simulink library "cpcAux"  (R2016a)
settings: Solver=ode45  StartTime=0.0  StopTime=10.0  RelTol=1e-3
undefined symbols (not defined in the file): DiscIntNeverNeededParam, sMP
libraries: simulink x16, cpcAux x8
(part 1 of 2)
settings Model: Creator=lzaimog  LastModifiedBy=PLOCH37
settings DataIOCC: LimitDataPoints=on
settings DebuggingCC: AllowSymbolicDim=off

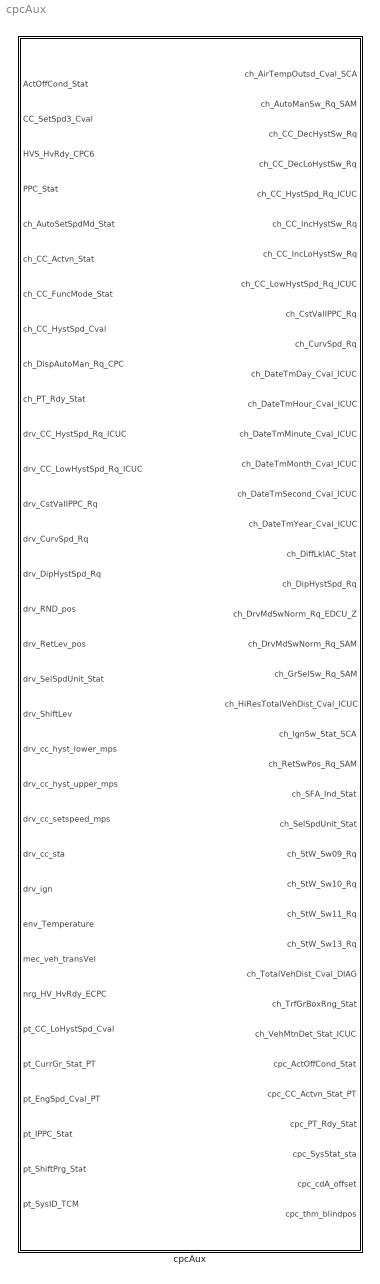
== system cpcAux ==
  cpcAux : Subsystem  TreatAsAtomicUnit=on  SystemSampleTime=0.1  mask{bShiftManual=sMP.ctrl.cpcAux.bShiftManual, s_shift_wait=sMP.ctrl.cpcAux.s_shift_wait, kmh_upshift=sMP.ctrl.cpcAux.kmh_upshift, kmh_downshift=sMP.ctrl.cpcAux.kmh_downshift, ShiftPrg=sMP.ctrl.cpcAux.ShiftPrg, CCFunc=sMP.ctrl.cpcAux.CCFunc, bCCbyPPC=sMP.ctrl.cpcAux.bCCbyPPC, x_id=sMP.ctrl.cpcAux.tfc_id, x_n=sMP.ctrl.cpcAux.tfc_gear, x_trqDistr=sMP.ctrl.cpcAux.tfc_trqDistribution, cdA_offset_sta=sMP.ctrl.cpcAux.cdA_offset_sta, cdA_offset_m2=sMP.ctrl.cpcAux.cdA_offset_m2, DateTmYear=sMP.ctrl.cpcAux.out.ch_DateTmYear_Cval_ICUC, DateTmMonth=sMP.ctrl.cpcAux.out.ch_DateTmMonth_Cval_ICUC, DateTmDay=sMP.ctrl.cpcAux.out.ch_DateTmDay_Cval_ICUC, DateTmHour=sMP.ctrl.cpcAux.out.ch_DateTmHour_Cval_ICUC, DateTmMinute=sMP.ctrl.cpcAux.out.ch_DateTmMinute_Cval_ICUC, DateTmSecond=sMP.ctrl.cpcAux.out.ch_DateTmSecond_Cval_ICUC}
      mask prompts: bShiftManual "Manual Shift [0,1]"; s_shift_wait "Wait Time between Shift [s]"; kmh_upshift "Upshift Speed [km/h]"; kmh_downshift "Downshift Speed [km/h]"; ShiftPrg "Drive program set by driver"; CCFunc "Function Mode [-]"; bCCbyPPC "CC controlled by IPPC [0,1]"; x_id "Type [-]"; x_n "Gear [-]"; x_trqDistr "Torque Distribution [%] (1x2)"; cdA_offset_sta "Blind position [-]"; cdA_offset_m2 "cd*A offset [m²]"; DateTmYear "Year"; DateTmMonth "Month"; DateTmDay "Day"; DateTmHour "Hour"; DateTmMinute "Minute"; DateTmSecond "Second"
      mask DialogControl DescTextVar Prompt: ICUC, SAM, ...

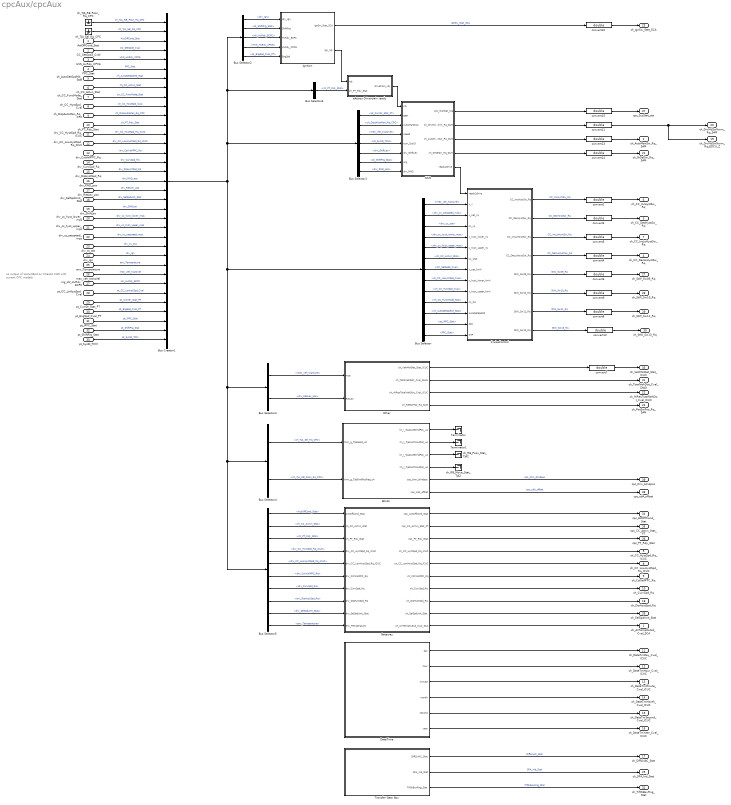
== system cpcAux/cpcAux ==
  note: no output of LoHystSpd on Chassis CAN
      | with current CPC models
  ActOffCond_Stat : Inport  OutDataTypeStr=double
  CC_SetSpd3_Cval : Inport  Port=2  OutDataTypeStr=double
  HVS_HvRdy_CPC6 : Inport  Port=3  OutDataTypeStr=double
  PPC_Stat : Inport  Port=4  OutDataTypeStr=double
  ch_AutoSetSpdMd_Stat : Inport  Port=5  OutDataTypeStr=double
  ch_CC_Actvn_Stat : Inport  Port=6  OutDataTypeStr=double
  ch_CC_FuncMode_Stat : Inport  Port=7  OutDataTypeStr=double
  ch_CC_HystSpd_Cval : Inport  Port=8  OutDataTypeStr=double
  ch_DispAutoMan_Rq_CPC : Inport  Port=9  OutDataTypeStr=double
  ch_PT_Rdy_Stat : Inport  Port=10  OutDataTypeStr=double
  drv_CC_HystSpd_Rq_ICUC : Inport  Port=11  OutDataTypeStr=double
  drv_CC_LowHystSpd_Rq_ICUC : Inport  Port=12  OutDataTypeStr=double
  drv_CstValIPPC_Rq : Inport  Port=13  OutDataTypeStr=double
  drv_CurvSpd_Rq : Inport  Port=14  OutDataTypeStr=double
  drv_DipHystSpd_Rq : Inport  Port=15  OutDataTypeStr=double
  drv_RND_pos : Inport  Port=16  OutDataTypeStr=double
  drv_RetLev_pos : Inport  Port=17  OutDataTypeStr=double
  drv_SelSpdUnit_Stat : Inport  Port=18  OutDataTypeStr=double
  drv_ShiftLev : Inport  Port=19  OutDataTypeStr=double
  drv_cc_hyst_lower_mps : Inport  Port=20  OutDataTypeStr=double
  drv_cc_hyst_upper_mps : Inport  Port=21  OutDataTypeStr=double
  drv_cc_setspeed_mps : Inport  Port=22  OutDataTypeStr=double
  drv_cc_sta : Inport  Port=23  OutDataTypeStr=double
  drv_ign : Inport  Port=24  OutDataTypeStr=double
  env_Temperature : Inport  Port=25  OutDataTypeStr=double
  mec_veh_transVel : Inport  Port=26  OutDataTypeStr=double
  nrg_HV_HvRdy_ECPC : Inport  Port=27  OutDataTypeStr=double
  pt_CC_LoHystSpd_Cval : Inport  Port=28  OutDataTypeStr=double
  pt_CurrGr_Stat_PT : Inport  Port=29  OutDataTypeStr=double
  pt_EngSpd_Cval_PT : Inport  Port=30  OutDataTypeStr=double
  pt_IPPC_Stat : Inport  Port=31  OutDataTypeStr=double
  pt_ShiftPrg_Stat : Inport  Port=32  OutDataTypeStr=double
  pt_SysID_TCM : Inport  Port=33  OutDataTypeStr=double
  Blinds : Subsystem  mask{cdA_offset_sta=cdA_offset_sta, cdA_offset_m2=cdA_offset_m2}
      mask prompts: cdA_offset_sta "Blind position [-]"; cdA_offset_m2 "cd*A offset [m²]"
      mask help:
      | Blind position [-]:
      | 0 - both open
      | 1 - bumper open, grill closed
      | 2 - bumper closed, grill open
      | 3 - both closed
  Bus Creator1 : BusCreator  Inputs=35
  Bus Selector : BusSelector  OutputSignals=mec_veh_transVel,drv_cc_setspeed_mps,drv_cc_sta,drv_cc_hyst_lower_mps,drv_cc_hyst_upper_mps,ch_CC_Actvn_Stat,CC_SetSpd3_Cval,pt_CC_LoHystSpd_Cval,ch_CC_HystSpd_Cval,ch_CC_FuncMode_Stat,ch_AutoSetSpdMd_Stat,pt_IPPC_Stat,PPC_Stat
  Bus Selector1 : BusSelector  OutputSignals=pt_CurrGr_Stat_PT,ch_DispAutoMan_Rq_CPC,mec_veh_transVel,pt_SysID_TCM,drv_ShiftLev,pt_ShiftPrg_Stat,drv_RND_pos
  Bus Selector2 : BusSelector  OutputSignals=drv_ign,pt_ShiftPrg_Stat,HV_HvRdy_ECPC,HVS_HvRdy_CPC6,pt_EngSpd_Cval_PT
  Bus Selector3 : BusSelector  OutputSignals=mec_veh_transVel,drv_RetLev_pos
  Bus Selector4 : BusSelector  OutputSignals=ch_TJA_Sel_Rq_CPC,ch_TJA_RB_Posn_Rq_CPC
  Bus Selector5 : BusSelector  OutputSignals=ActOffCond_Stat,ch_CC_Actvn_Stat,ch_PT_Rdy_Stat,drv_CC_HystSpd_Rq_ICUC,drv_CC_LowHystSpd_Rq_ICUC,drv_CstValIPPC_Rq,drv_CurvSpd_Rq,drv_DipHystSpd_Rq,drv_SelSpdUnit_Stat,env_Temperature
  Bus Selector6 : BusSelector  OutputSignals=ch_PT_Rdy_Stat
  CruiseControl : Subsystem
  DateTime : Subsystem  mask{DateTmSecond=DateTmSecond, DateTmMinute=DateTmMinute, DateTmHour=DateTmHour, DateTmDay=DateTmDay, DateTmMonth=DateTmMonth, DateTmYear=DateTmYear}
      mask prompts: DateTmSecond "ICUC_DateTmSecond [s]"; DateTmMinute "ICUC_DateTmMinute [min]"; DateTmHour "ICUC_DateTmHour [h]"; DateTmDay "ICUC_DateTmDay [day]"; DateTmMonth "ICUC_DateTmMonth [month]"; DateTmYear "ICUC_DateTmYear [year]"
  Gateway : Subsystem
  Ignition : Subsystem
  Other : Subsystem
  Shift : Subsystem
  Terminator : Terminator
  Terminator1 : Terminator
  Transfer Gear Box : Subsystem
  ch_RB_Move_Stat_TJA2 : Terminator
  ch_RB_Posn_Stat_TJA2 : Terminator
  ch_TJA_RB_Posn_Rq_CPC : Ground
  ch_TJA_Sel_Rq_CPC : Ground
  convert{2..15} (14 alike) : DataTypeConversion  OutDataTypeStr=double  SaturateOnIntegerOverflow=on  RndMeth=Zero
  eActros Drivertrain ready : Subsystem
  ch_AirTempOutsd_Cval_SCA : Outport
  ch_AutoManSw_Rq_SAM : Outport  Port=2
  ch_CC_DecHystSw_Rq : Outport  Port=3
  ch_CC_DecLoHystSw_Rq : Outport  Port=4
  ch_CC_HystSpd_Rq_ICUC : Outport  Port=5
  ch_CC_IncHystSw_Rq : Outport  Port=6
  ch_CC_IncLoHystSw_Rq : Outport  Port=7
  ch_CC_LowHystSpd_Rq_ICUC : Outport  Port=8
  ch_CstValIPPC_Rq : Outport  Port=9
  ch_CurvSpd_Rq : Outport  Port=10
  ch_DateTmDay_Cval_ICUC : Outport  Port=11
  ch_DateTmHour_Cval_ICUC : Outport  Port=12
  ch_DateTmMinute_Cval_ICUC : Outport  Port=13
  ch_DateTmMonth_Cval_ICUC : Outport  Port=14
  ch_DateTmSecond_Cval_ICUC : Outport  Port=15
  ch_DateTmYear_Cval_ICUC : Outport  Port=16
  ch_DiffLkIAC_Stat : Outport  Port=17
  ch_DipHystSpd_Rq : Outport  Port=18
  ch_DrvMdSwNorm_Rq_EDCU_Z : Outport  Port=19
  ch_DrvMdSwNorm_Rq_SAM : Outport  Port=20
  ch_GrSelSw_Rq_SAM : Outport  Port=21
  ch_HiResTotalVehDist_Cval_ICUC : Outport  Port=22
  ch_IgnSw_Stat_SCA : Outport  Port=23
  ch_RetSwPos_Rq_SAM : Outport  Port=24
  ch_SFA_Ind_Stat : Outport  Port=25
  ch_SelSpdUnit_Stat : Outport  Port=26
  ch_StW_Sw09_Rq : Outport  Port=27
  ch_StW_Sw10_Rq : Outport  Port=28
  ch_StW_Sw11_Rq : Outport  Port=29
  ch_StW_Sw13_Rq : Outport  Port=30
  ch_TotalVehDist_Cval_DIAG : Outport  Port=31
  ch_TrfGrBoxRng_Stat : Outport  Port=32
  ch_VehMtnDet_Stat_ICUC : Outport  Port=33
  cpc_ActOffCond_Stat : Outport  Port=34
  cpc_CC_Actvn_Stat_PT : Outport  Port=35
  cpc_PT_Rdy_Stat : Outport  Port=36
  cpc_SysStat_sta : Outport  Port=37
  cpc_cdA_offset : Outport  Port=38
  cpc_thm_blindpos : Outport  Port=39
  wires:
  Gateway/1(cpc_ActOffCond_Stat) -> cpc_ActOffCond_Stat/1
  Bus Selector5/1 -> Gateway/1(ActOffCond_Stat)  "<ActOffCond_Stat>"
  ActOffCond_Stat/1 -> Bus Creator1/3  "ActOffCond_Stat"
  Bus Selector/13 -> CruiseControl/14(CTP)  "<PPC_Stat>"
  PPC_Stat/1 -> Bus Creator1/6  "PPC_Stat"
  Bus Selector2/4 -> Ignition/4(HvRdy_CPC6)  "<HVS_HvRdy_CPC6>"
  Bus Selector2/3 -> Ignition/3(HvRdy_ECPC)  "<HV_HvRdy_ECPC>"
  Bus Selector2/2 -> Ignition/2(ShiftPrg)  "<pt_ShiftPrg_Stat>"
  nrg_HV_HvRdy_ECPC/1 -> Bus Creator1/29  "HV_HvRdy_ECPC"
  HVS_HvRdy_CPC6/1 -> Bus Creator1/5  "HVS_HvRdy_CPC6"
  Bus Selector1/7 -> Shift/8(drv_RND)  "<drv_RND_pos>"
  drv_RND_pos/1 -> Bus Creator1/18  "drv_RND_pos"
  Other/3(ch_HiResTotalVehDist_Cval_ICUC) -> ch_HiResTotalVehDist_Cval_ICUC/1
  Bus Selector1/6 -> Shift/7(prg)  "<pt_ShiftPrg_Stat>"
  pt_ShiftPrg_Stat/1 -> Bus Creator1/34  "pt_ShiftPrg_Stat"
  ch_TJA_Sel_Rq_CPC/1 -> Bus Creator1/2  "ch_TJA_Sel_Rq_CPC"
  ch_TJA_RB_Posn_Rq_CPC/1 -> Bus Creator1/1  "ch_TJA_RB_Posn_Rq_CPC"
  drv_RetLev_pos/1 -> Bus Creator1/19  "drv_RetLev_pos"
  ch_AutoSetSpdMd_Stat/1 -> Bus Creator1/7  "ch_AutoSetSpdMd_Stat"
  drv_ign/1 -> Bus Creator1/26  "drv_ign"
  env_Temperature/1 -> Bus Creator1/27  "env_Temperature"
  drv_CC_HystSpd_Rq_ICUC/1 -> Bus Creator1/13  "drv_CC_HystSpd_Rq_ICUC"
  drv_cc_hyst_lower_mps/1 -> Bus Creator1/22  "drv_cc_hyst_lower_mps"
  drv_SelSpdUnit_Stat/1 -> Bus Creator1/20  "drv_SelSpdUnit_Stat"
  ch_DispAutoMan_Rq_CPC/1 -> Bus Creator1/11  "ch_DispAutoMan_Rq_CPC"
  ch_CC_FuncMode_Stat/1 -> Bus Creator1/9  "ch_CC_FuncMode_Stat"
  pt_CC_LoHystSpd_Cval/1 -> Bus Creator1/30  "pt_CC_LoHystSpd_Cval"
  drv_CstValIPPC_Rq/1 -> Bus Creator1/15  "drv_CstValIPPC_Rq"
  ch_CC_Actvn_Stat/1 -> Bus Creator1/8  "ch_CC_Actvn_Stat"
  drv_DipHystSpd_Rq/1 -> Bus Creator1/17  "drv_DipHystSpd_Rq"
  drv_cc_hyst_upper_mps/1 -> Bus Creator1/23  "drv_cc_hyst_upper_mps"
  pt_SysID_TCM/1 -> Bus Creator1/35  "pt_SysID_TCM"
  pt_EngSpd_Cval_PT/1 -> Bus Creator1/32  "pt_EngSpd_Cval_PT"
  drv_cc_sta/1 -> Bus Creator1/25  "drv_cc_sta"
  drv_CC_LowHystSpd_Rq_ICUC/1 -> Bus Creator1/14  "drv_CC_LowHystSpd_Rq_ICUC"
  pt_IPPC_Stat/1 -> Bus Creator1/33  "pt_IPPC_Stat"
  drv_cc_setspeed_mps/1 -> Bus Creator1/24  "drv_cc_setspeed_mps"
  drv_ShiftLev/1 -> Bus Creator1/21  "drv_ShiftLev"
  mec_veh_transVel/1 -> Bus Creator1/28  "mec_veh_transVel"
  pt_CurrGr_Stat_PT/1 -> Bus Creator1/31  "pt_CurrGr_Stat_PT"
  CC_SetSpd3_Cval/1 -> Bus Creator1/4  "CC_SetSpd3_Cval"
  drv_CurvSpd_Rq/1 -> Bus Creator1/16  "drv_CurvSpd_Rq"
  ch_CC_HystSpd_Cval/1 -> Bus Creator1/10  "ch_CC_HystSpd_Cval"
  ch_PT_Rdy_Stat/1 -> Bus Creator1/12  "ch_PT_Rdy_Stat"
  Other/4(ch_RetSwPos_Rq_SAM) -> ch_RetSwPos_Rq_SAM/1
  Bus Selector3/2 -> Other/2(RetLev)  "<drv_RetLev_pos>"
  Bus Selector1/2 -> Shift/3(AutoManDisp)  "<ch_DispAutoMan_Rq_CPC>"
  Transfer Gear Box/1(DiffLkIAC_Stat) -> ch_DiffLkIAC_Stat/1  "DiffLkIAC_Stat"
  Transfer Gear Box/2(SFA_Ind_Stat) -> ch_SFA_Ind_Stat/1  "SFA_Ind_Stat"
  Transfer Gear Box/3(TrfGrBoxRng_Stat) -> ch_TrfGrBoxRng_Stat/1  "TrfGrBoxRng_Stat"
  Gateway/6(ch_CstValIPPC_Rq) -> ch_CstValIPPC_Rq/1
  Gateway/7(ch_CurvSpd_Rq) -> ch_CurvSpd_Rq/1
  Bus Selector5/7 -> Gateway/7(drv_CurvSpd_Rq)  "<drv_CurvSpd_Rq>"
  Bus Selector5/6 -> Gateway/6(drv_CstValIPPC_Rq)  "<drv_CstValIPPC_Rq>"
  Bus Selector/12 -> CruiseControl/13(PPC)  "<pt_IPPC_Stat>"
  Bus Selector/11 -> CruiseControl/12(AutoSetSpdMd)  "<ch_AutoSetSpdMd_Stat>"
  Gateway/3(cpc_PT_Rdy_Stat) -> cpc_PT_Rdy_Stat/1
  Bus Selector5/3 -> Gateway/3(ch_PT_Rdy_Stat)  "<ch_PT_Rdy_Stat>"
  Gateway/2(cpc_CC_Actvn_Stat_PT) -> cpc_CC_Actvn_Stat_PT/1
  Bus Selector5/2 -> Gateway/2(ch_CC_Actvn_Stat)  "<ch_CC_Actvn_Stat>"
  Bus Selector2/1 -> Ignition/1(drv_ign)  "<drv_ign>"
  convert15/1 -> cpc_SysStat_sta/1
  convert14/1 -> ch_GrSelSw_Rq_SAM/1
  convert13/1 -> ch_AutoManSw_Rq_SAM/1
  Shift/3(ch_AutoManSw_Rq_SAM) -> convert13/1
  Shift/4(ch_GrSelSw_Rq_SAM) -> convert14/1
  Bus Selector1/5 -> Shift/6(drv_ShiftLev)  "<drv_ShiftLev>"
  Shift/5(ready2drive) -> CruiseControl/1(ready2drive)
  eActros Drivertrain ready/1(drivetrain_rdy) -> Shift/1(rdy)
  Bus Selector6/1 -> eActros Drivertrain ready/2(ch_PT_Rdy_Stat)  "<ch_PT_Rdy_Stat>"
  Ignition/2(ign_rdy) -> eActros Drivertrain ready/1(rdy)
  Bus Selector1/4 -> Shift/5(tcm_SysID)  "<pt_SysID_TCM>"
  Other/2(ch_TotalVehDist_Cval_DIAG) -> ch_TotalVehDist_Cval_DIAG/1
  convert12/1 -> ch_StW_Sw13_Rq/1
  Bus Selector5/5 -> Gateway/5(drv_CC_LowHystSpd_Rq_ICUC)  "<drv_CC_LowHystSpd_Rq_ICUC>"
  Bus Selector5/4 -> Gateway/4(drv_CC_HystSpd_Rq_ICUC)  "<drv_CC_HystSpd_Rq_ICUC>"
  Bus Selector/1 -> CruiseControl/2(v_v)  "<mec_veh_transVel>"
  CruiseControl/1(CC_IncHystSw_Rq) -> convert2/1  "CC_IncHystSw_Rq"
  CruiseControl/2(CC_DecHystSw_Rq) -> convert3/1  "CC_DecHystSw_Rq"
  CruiseControl/3(CC_IncLoHystSw_Rq) -> convert5/1  "CC_IncLoHystSw_Rq"
  CruiseControl/4(CC_DecLoHystSw_Rq) -> convert4/1  "CC_DecLoHystSw_Rq"
  CruiseControl/5(StW_Sw09_Rq) -> convert6/1  "StW_Sw09_Rq"
  CruiseControl/6(StW_Sw10_Rq) -> convert9/1  "StW_Sw10_Rq"
  CruiseControl/7(StW_Sw11_Rq) -> convert8/1  "StW_Sw11_Rq"
  CruiseControl/8(StW_Sw13_Rq) -> convert12/1  "StW_Sw13_Rq"
  Ignition/1(IgnSw_Stat_SCA) -> convert10/1  "IgnSw_Stat_SCA"
  Gateway/4(ch_CC_HystSpd_Rq_ICUC) -> ch_CC_HystSpd_Rq_ICUC/1
  Gateway/5(ch_CC_LowHystSpd_Rq_ICUC) -> ch_CC_LowHystSpd_Rq_ICUC/1
  Other/1(ch_VehMtnDet_Stat_ICUC) -> convert7/1
  DateTime/6(year) -> ch_DateTmYear_Cval_ICUC/1
  DateTime/4(month) -> ch_DateTmMonth_Cval_ICUC/1
  DateTime/5(second) -> ch_DateTmSecond_Cval_ICUC/1
  DateTime/1(day) -> ch_DateTmDay_Cval_ICUC/1
  DateTime/2(hour) -> ch_DateTmHour_Cval_ICUC/1
  DateTime/3(minute) -> ch_DateTmMinute_Cval_ICUC/1
  Gateway/10(ch_AirTempOutsd_Cval_SCA) -> ch_AirTempOutsd_Cval_SCA/1
  Gateway/8(ch_DipHystSpd_Rq) -> ch_DipHystSpd_Rq/1
  Gateway/9(ch_SelSpdUnit_Stat) -> ch_SelSpdUnit_Stat/1
  Bus Selector2/5 -> Ignition/5(EngSpd)  "<pt_EngSpd_Cval_PT>"
  Bus Selector/2 -> CruiseControl/3(v_set_rq)  "<drv_cc_setspeed_mps>"
  Bus Selector/3 -> CruiseControl/4(cc_rq)  "<drv_cc_sta>"
  Bus Selector/4 -> CruiseControl/5(v_hyst_lower_rq)  "<drv_cc_hyst_lower_mps>"
  Bus Selector/5 -> CruiseControl/6(v_hyst_upper_rq)  "<drv_cc_hyst_upper_mps>"
  Bus Selector/6 -> CruiseControl/7(cc_stat)  "<ch_CC_Actvn_Stat>"
  Bus Selector/7 -> CruiseControl/8(v_set_kmh)  "<CC_SetSpd3_Cval>"
  Bus Selector/8 -> CruiseControl/9(v_hyst_lower_kmh)  "<pt_CC_LoHystSpd_Cval>"
  Bus Selector/9 -> CruiseControl/10(v_hyst_upper_kmh)  "<ch_CC_HystSpd_Cval>"
  Bus Selector/10 -> CruiseControl/11(cc_fun)  "<ch_CC_FuncMode_Stat>"
  Bus Selector3/1 -> Other/1(mps)  "<mec_veh_transVel>"
  Bus Selector1/1 -> Shift/2(gear)  "<pt_CurrGr_Stat_PT>"
  Bus Selector1/3 -> Shift/4(speed)  "<mec_veh_transVel>"
  Shift/1(cpc_SysStat_sta) -> convert15/1
  Shift/2(ch_DrvMdSwNorm_Rq_SAM) -> convert11/1
  Bus Selector5/8 -> Gateway/8(drv_DipHystSpd_Rq)  "<drv_DipHystSpd_Rq>"
  Bus Selector5/9 -> Gateway/9(drv_SelSpdUnit_Stat)  "<drv_SelSpdUnit_Stat>"
  Bus Selector5/10 -> Gateway/10(env_Temperature)  "<env_Temperature>"
  Blinds/5(cpc_thm_blindpos) -> cpc_thm_blindpos/1  "cpc_thm_blindpos"
  Blinds/6(cpc_cdA_offset) -> cpc_cdA_offset/1  "cpc_cdA_offset"
  Blinds/2(lin_i_Tja1ActMovStat_u4) -> Terminator1/1
  Blinds/1(lin_i_Tja1ActBlindPos_u4) -> Terminator/1
  Bus Creator1/1 -> Bus Selector1/1, Bus Selector6/1, Bus Selector2/1, Bus Selector/1, Bus Selector3/1, Bus Selector4/1, Bus Selector5/1
  Blinds/3(lin_i_Tja2ActBlindPos_u4) -> ch_RB_Posn_Stat_TJA2/1
  Blinds/4(lin_i_Tja2ActMovStat_u4) -> ch_RB_Move_Stat_TJA2/1
  Bus Selector4/1 -> Blinds/1(thm_g_TjaReqId_u2)  "<ch_TJA_Sel_Rq_CPC>"
  Bus Selector4/2 -> Blinds/2(thm_g_TjaBlindPosReq_u4)  "<ch_TJA_RB_Posn_Rq_CPC>"
  convert7/1 -> ch_VehMtnDet_Stat_ICUC/1
  convert2/1 -> ch_CC_IncHystSw_Rq/1
  convert3/1 -> ch_CC_DecHystSw_Rq/1
  convert5/1 -> ch_CC_IncLoHystSw_Rq/1
  convert4/1 -> ch_CC_DecLoHystSw_Rq/1
  convert6/1 -> ch_StW_Sw09_Rq/1
  convert9/1 -> ch_StW_Sw10_Rq/1
  convert8/1 -> ch_StW_Sw11_Rq/1
  convert10/1 -> ch_IgnSw_Stat_SCA/1
  convert11/1 -> ch_DrvMdSwNorm_Rq_EDCU_Z/1, ch_DrvMdSwNorm_Rq_SAM/1

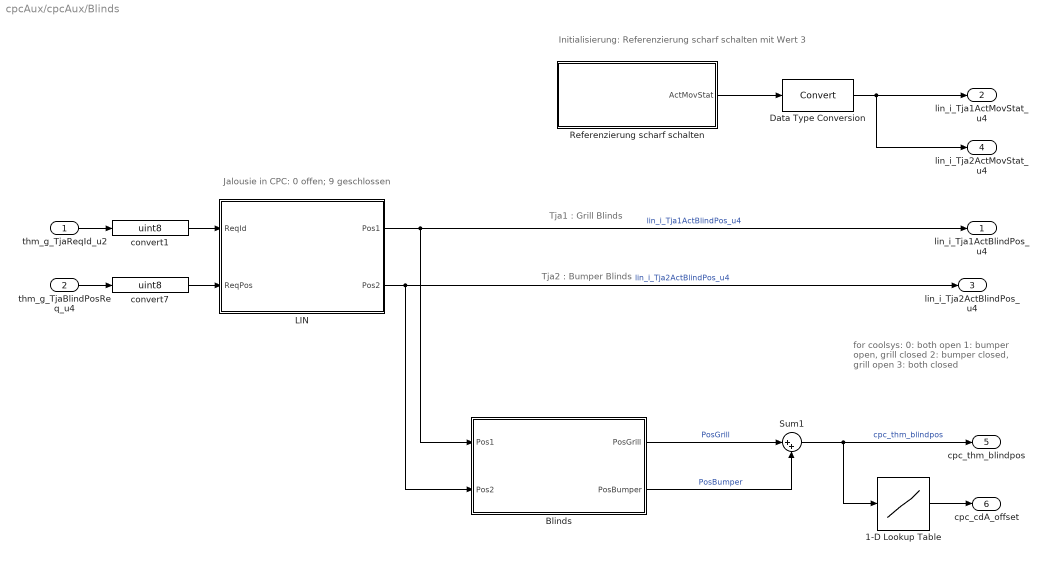
== system cpcAux/cpcAux/Blinds ==
  note: Initialisierung: Referenzierung scharf schalten mit Wert 3
  note: Jalousie in CPC: 0 offen; 9 geschlossen
  note: Tja1 : Grill Blinds
  note: Tja2 : Bumper Blinds
  note: for coolsys:
      | 0: both open
      | 1: bumper open, grill closed
      | 2: bumper closed, grill open
      | 3: both closed
  thm_g_TjaReqId_u2 : Inport
  thm_g_TjaBlindPosReq_u4 : Inport  Port=2
  1-D Lookup Table : Lookup_n-D  NumberOfTableDimensions=1  BreakpointsForDimension1=cdA_offset_sta  Table=cdA_offset_m2  InternalRulePriority=Speed  RndMeth=Simplest  InputSameDT=on
  Blinds : Stateflow chart  TreatAsAtomicUnit=on
  Data Type Conversion : DataTypeConversion
  LIN : Stateflow chart  TreatAsAtomicUnit=on
  Referenzierung scharf schalten : Subsystem
  Sum1 : Sum  Inputs=|++
  convert1 : DataTypeConversion  OutDataTypeStr=uint8  SaturateOnIntegerOverflow=on  RndMeth=Zero
  convert7 : DataTypeConversion  OutDataTypeStr=uint8  SaturateOnIntegerOverflow=on  RndMeth=Zero
  lin_i_Tja1ActBlindPos_u4 : Outport
  lin_i_Tja1ActMovStat_u4 : Outport  Port=2
  lin_i_Tja2ActBlindPos_u4 : Outport  Port=3
  lin_i_Tja2ActMovStat_u4 : Outport  Port=4
  cpc_thm_blindpos : Outport  Port=5
  cpc_cdA_offset : Outport  Port=6
  wires:
  LIN/2(Pos2) -> lin_i_Tja2ActBlindPos_u4/1, Blinds/2(Pos2)  "lin_i_Tja2ActBlindPos_u4"
  LIN/1(Pos1) -> lin_i_Tja1ActBlindPos_u4/1, Blinds/1(Pos1)  "lin_i_Tja1ActBlindPos_u4"
  thm_g_TjaBlindPosReq_u4/1 -> convert7/1
  thm_g_TjaReqId_u2/1 -> convert1/1
  Blinds/2(PosBumper) -> Sum1/2  "PosBumper"
  Blinds/1(PosGrill) -> Sum1/1  "PosGrill"
  Data Type Conversion/1 -> lin_i_Tja2ActMovStat_u4/1, lin_i_Tja1ActMovStat_u4/1
  Referenzierung scharf schalten/1(ActMovStat) -> Data Type Conversion/1
  Sum1/1 -> cpc_thm_blindpos/1, 1-D Lookup Table/1  "cpc_thm_blindpos"
  1-D Lookup Table/1 -> cpc_cdA_offset/1
  convert7/1 -> LIN/2(ReqPos)
  convert1/1 -> LIN/1(ReqId)

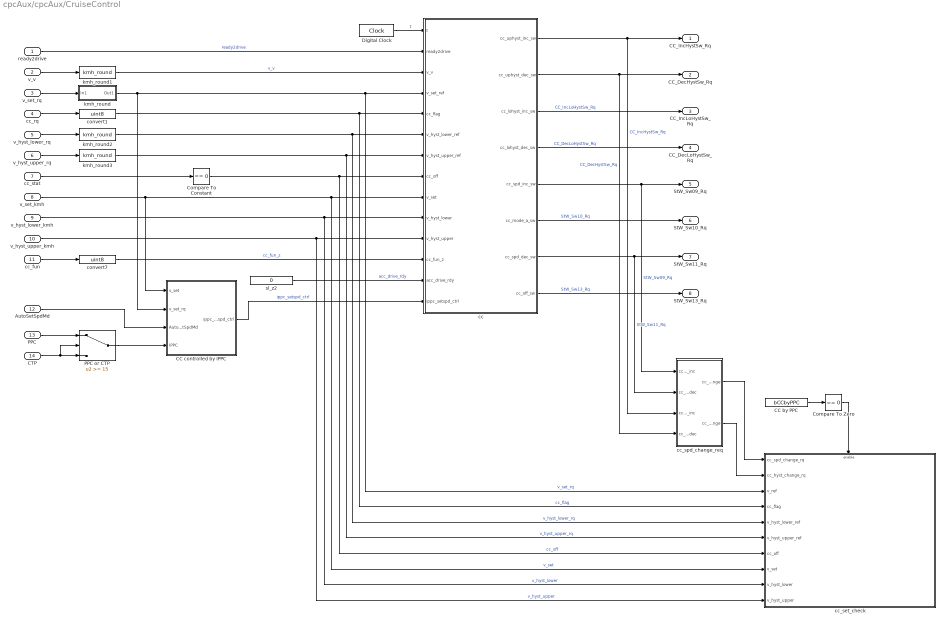
== system cpcAux/cpcAux/CruiseControl ==
  ready2drive : Inport
  v_v : Inport  Port=2
  v_set_rq : Inport  Port=3
  cc_rq : Inport  Port=4
  v_hyst_lower_rq : Inport  Port=5
  v_hyst_upper_rq : Inport  Port=6
  cc_stat : Inport  Port=7
  v_set_kmh : Inport  Port=8
  v_hyst_lower_kmh : Inport  Port=9
  v_hyst_upper_kmh : Inport  Port=10
  cc_fun : Inport  Port=11
  AutoSetSpdMd : Inport  Port=12
  PPC : Inport  Port=13
  CTP : Inport  Port=14
  CC by PPC : Constant  Value=bCCbyPPC
  CC controlled by IPPC : Subsystem
  Compare To Constant : simulink/Logic and Bit Operations/Compare To Constant  relop===  const=0  OutDataTypeStr=uint8
  Compare To Zero : simulink/Logic and Bit Operations/Compare To Zero  relop===  OutDataTypeStr=boolean
  Digital Clock : DigitalClock  SampleTime=-1
  PPC or CTP : Switch  Threshold=15
  cc : Stateflow chart  TreatAsAtomicUnit=on
  cc_set_check : Subsystem
  cc_spd_change_req : Subsystem
  convert1 : DataTypeConversion  OutDataTypeStr=uint8  SaturateOnIntegerOverflow=on  RndMeth=Zero
  convert7 : DataTypeConversion  OutDataTypeStr=uint8  SaturateOnIntegerOverflow=on  RndMeth=Zero
  kmh_round : Subsystem  mask(Speed converter){resolution=0.5}
      mask help:
      | Convert m/s to km/h and
      | Round values to defined resolution
      settings: AttributesFormatString=%<resolution>
      mask Display: disp('m/s to km/h\n and round')
  kmh_round1 : cpcAux/cpcAux/CruiseControl/kmh_round  resolution=0.1
      settings: AttributesFormatString=%<resolution>
  kmh_round2 : cpcAux/cpcAux/CruiseControl/kmh_round  resolution=1
      settings: AttributesFormatString=%<resolution>
  kmh_round3 : cpcAux/cpcAux/CruiseControl/kmh_round  resolution=1
      settings: AttributesFormatString=%<resolution>
  sl_z2 : Constant  Value=0  OutDataTypeStr=Inherit: Inherit via back propagation
  CC_IncHystSw_Rq : Outport
  CC_DecHystSw_Rq : Outport  Port=2
  CC_IncLoHystSw_Rq : Outport  Port=3
  CC_DecLoHystSw_Rq : Outport  Port=4
  StW_Sw09_Rq : Outport  Port=5
  StW_Sw10_Rq : Outport  Port=6
  StW_Sw11_Rq : Outport  Port=7
  StW_Sw13_Rq : Outport  Port=8
  wires:
  PPC or CTP/1 -> CC controlled by IPPC/4(IPPC)
  CTP/1 -> PPC or CTP/3, PPC or CTP/2
  Compare To Zero/1 -> cc_set_check/Enable
  CC by PPC/1 -> Compare To Zero/1
  CC controlled by IPPC/1(ippc_setspd_ctrl) -> cc/14(ippc_setspd_ctrl)  "ippc_setspd_ctrl"
  PPC/1 -> PPC or CTP/1
  AutoSetSpdMd/1 -> CC controlled by IPPC/3(AutoSetSpdMd)
  cc_spd_change_req/2(cc_hyst_change) -> cc_set_check/2(cc_hyst_change_rq)
  kmh_round1/1 -> cc/3(v_v)  "v_v"
  convert1/1 -> cc/5(cc_flag), cc_set_check/4(cc_flag)  "cc_flag"
  cc_spd_change_req/1(cc_spd_change) -> cc_set_check/1(cc_spd_change_rq)
  v_hyst_upper_kmh/1 -> cc/11(v_hyst_upper), cc_set_check/10(v_hyst_upper)  "v_hyst_upper"
  v_hyst_lower_kmh/1 -> cc/10(v_hyst_lower), cc_set_check/9(v_hyst_lower)  "v_hyst_lower"
  v_set_kmh/1 -> CC controlled by IPPC/1(v_set), cc/9(v_set), cc_set_check/8(v_set)  "v_set"
  Compare To Constant/1 -> cc_set_check/7(cc_off), cc/8(cc_off)  "cc_off"
  kmh_round3/1 -> cc/7(v_hyst_upper_ref), cc_set_check/6(v_hyst_upper_ref)  "v_hyst_upper_rq"
  kmh_round2/1 -> cc/6(v_hyst_lower_ref), cc_set_check/5(v_hyst_lower_ref)  "v_hyst_lower_rq"
  cc_rq/1 -> convert1/1
  Digital Clock/1 -> cc/1(t)  "t"
  v_v/1 -> kmh_round1/1
  ready2drive/1 -> cc/2(ready2drive)  "ready2drive"
  sl_z2/1 -> cc/13(acc_drive_rdy)  "acc_drive_rdy"
  v_set_rq/1 -> kmh_round/1(In1)
  v_hyst_lower_rq/1 -> kmh_round2/1
  cc/1(cc_uphyst_inc_sw) -> cc_spd_change_req/3(cc_hyst_inc), CC_IncHystSw_Rq/1  "CC_IncHystSw_Rq"
  v_hyst_upper_rq/1 -> kmh_round3/1
  cc/2(cc_uphyst_dec_sw) -> cc_spd_change_req/4(cc_hyst_dec), CC_DecHystSw_Rq/1  "CC_DecHystSw_Rq"
  cc_fun/1 -> convert7/1
  cc/4(cc_lohyst_dec_sw) -> CC_DecLoHystSw_Rq/1  "CC_DecLoHystSw_Rq"
  cc/5(cc_spd_inc_sw) -> cc_spd_change_req/1(cc_spd_inc), StW_Sw09_Rq/1  "StW_Sw09_Rq"
  cc/7(cc_spd_dec_sw) -> cc_spd_change_req/2(cc_spc_dec), StW_Sw11_Rq/1  "StW_Sw11_Rq"
  cc/6(cc_mode_a_sw) -> StW_Sw10_Rq/1  "StW_Sw10_Rq"
  cc/8(cc_off_sw) -> StW_Sw13_Rq/1  "StW_Sw13_Rq"
  cc_stat/1 -> Compare To Constant/1
  cc/3(cc_lohyst_inc_sw) -> CC_IncLoHystSw_Rq/1  "CC_IncLoHystSw_Rq"
  kmh_round/1(Out1) -> CC controlled by IPPC/2(v_set_rq), cc/4(v_set_ref), cc_set_check/3(v_ref)  "v_set_rq"
  convert7/1 -> cc/12(cc_fun_z)  "cc_fun_z"

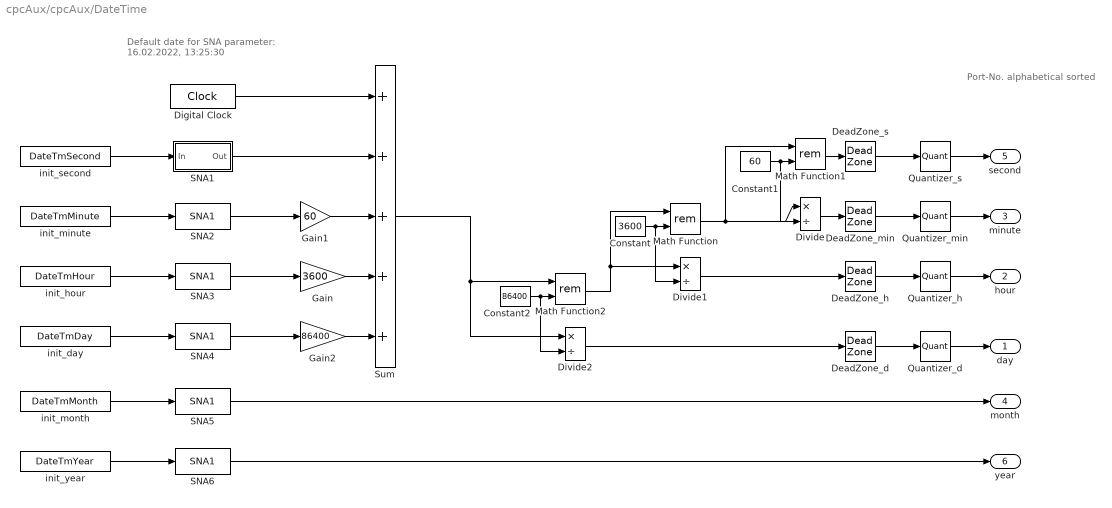
== system cpcAux/cpcAux/DateTime ==
  note: Default date for SNA parameter:
      | 16.02.2022, 13:25:30
  note: Port-No.
      | alphabetical
      | sorted
  Constant : Constant  Value=3600
  Constant1 : Constant  Value=60
  Constant2 : Constant  Value=86400
  DeadZone_d : DeadZone  SaturateOnIntegerOverflow=on
  DeadZone_h : DeadZone  SaturateOnIntegerOverflow=on
  DeadZone_min : DeadZone  SaturateOnIntegerOverflow=on
  DeadZone_s : DeadZone  SaturateOnIntegerOverflow=on
  Digital Clock : DigitalClock  SampleTime=-1
  Divide : Product  Inputs=*/
  Divide1 : Product  Inputs=*/
  Divide2 : Product  Inputs=*/
  Gain : Gain  Gain=3600
  Gain1 : Gain  Gain=60
  Gain2 : Gain  Gain=86400
  Math Function : Math  Operator=rem  SaturateOnIntegerOverflow=on
  Math Function1 : Math  Operator=rem  SaturateOnIntegerOverflow=on
  Math Function2 : Math  Operator=rem  SaturateOnIntegerOverflow=on
  Quantizer_d : Quantizer  QuantizationInterval=1
  Quantizer_h : Quantizer  QuantizationInterval=1
  Quantizer_min : Quantizer  QuantizationInterval=1
  Quantizer_s : Quantizer  QuantizationInterval=1
  SNA1 : Subsystem  mask{sna_max=59, sna_eq=30}
      mask prompts: sna_max "max value"; sna_eq "equivalent value"
      mask help: If value above max value, it will be replaced by equivalent value
      settings: AttributesFormatString=x > %<sna_max>: %<sna_eq>
  SNA2 : cpcAux/cpcAux/DateTime/SNA1  sna_max=59  sna_eq=25
      settings: AttributesFormatString=x > %<sna_max>: %<sna_eq>
  SNA3 : cpcAux/cpcAux/DateTime/SNA1  sna_max=23  sna_eq=13
      settings: AttributesFormatString=x > %<sna_max>: %<sna_eq>
  SNA4 : cpcAux/cpcAux/DateTime/SNA1  sna_max=31  sna_eq=16
      settings: AttributesFormatString=x > %<sna_max>: %<sna_eq>
  SNA5 : cpcAux/cpcAux/DateTime/SNA1  sna_max=12  sna_eq=2
      settings: AttributesFormatString=x > %<sna_max>: %<sna_eq>
  SNA6 : cpcAux/cpcAux/DateTime/SNA1  sna_max=2234  sna_eq=2022
      settings: AttributesFormatString=x > %<sna_max>: %<sna_eq>
  Sum : Sum  Inputs=5
  init_day : Constant  InitFcn=""  Value=DateTmDay
  init_hour : Constant  Value=DateTmHour
  init_minute : Constant  Value=DateTmMinute
  init_month : Constant  Value=DateTmMonth
  init_second : Constant  Value=DateTmSecond
  init_year : Constant  Value=DateTmYear
  day : Outport
  hour : Outport  Port=2
  minute : Outport  Port=3
  month : Outport  Port=4
  second : Outport  Port=5
  year : Outport  Port=6
  wires:
  Digital Clock/1 -> Sum/1
  init_hour/1 -> SNA3/1
  init_minute/1 -> SNA2/1
  init_second/1 -> SNA1/1(In)
  Gain1/1 -> Sum/3
  Gain/1 -> Sum/4
  Constant/1 -> Math Function/2, Divide1/2
  Constant1/1 -> Math Function1/2, Divide/2
  Math Function/1 -> Math Function1/1, Divide/1
  Math Function1/1 -> DeadZone_s/1
  Divide/1 -> DeadZone_min/1
  Divide1/1 -> DeadZone_h/1
  DeadZone_min/1 -> Quantizer_min/1
  DeadZone_s/1 -> Quantizer_s/1
  DeadZone_h/1 -> Quantizer_h/1
  Quantizer_s/1 -> second/1
  Quantizer_min/1 -> minute/1
  Quantizer_h/1 -> hour/1
  init_year/1 -> SNA6/1
  init_day/1 -> SNA4/1
  init_month/1 -> SNA5/1
  DeadZone_d/1 -> Quantizer_d/1
  Quantizer_d/1 -> day/1
  Constant2/1 -> Divide2/2, Math Function2/2
  Math Function2/1 -> Math Function/1, Divide1/1
  Sum/1 -> Math Function2/1, Divide2/1
  Gain2/1 -> Sum/5
  Divide2/1 -> DeadZone_d/1
  SNA1/1(Out) -> Sum/2
  SNA2/1 -> Gain1/1
  SNA3/1 -> Gain/1
  SNA4/1 -> Gain2/1
  SNA5/1 -> month/1
  SNA6/1 -> year/1

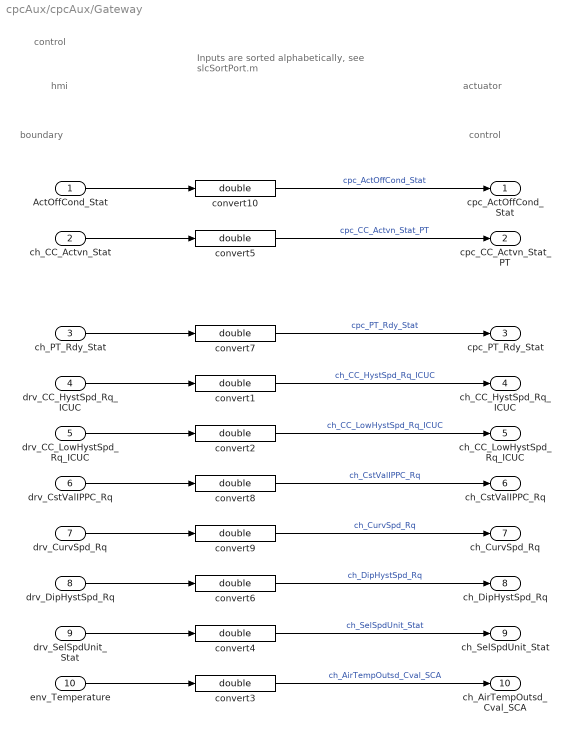
== system cpcAux/cpcAux/Gateway ==
  note: control
  note: actuator
  note: boundary
  note: hmi
  note: control
  note: Inputs are sorted
      | alphabetically,
      | see slcSortPort.m
  ActOffCond_Stat : Inport
  ch_CC_Actvn_Stat : Inport  Port=2
  ch_PT_Rdy_Stat : Inport  Port=3
  drv_CC_HystSpd_Rq_ICUC : Inport  Port=4
  drv_CC_LowHystSpd_Rq_ICUC : Inport  Port=5
  drv_CstValIPPC_Rq : Inport  Port=6
  drv_CurvSpd_Rq : Inport  Port=7
  drv_DipHystSpd_Rq : Inport  Port=8
  drv_SelSpdUnit_Stat : Inport  Port=9
  env_Temperature : Inport  Port=10
  convert{1..10} (10 alike) : DataTypeConversion  OutDataTypeStr=double  SaturateOnIntegerOverflow=on  RndMeth=Zero
  cpc_ActOffCond_Stat : Outport  Description=needed for driver to enable CC
      settings: AttributesFormatString=%<Description>
  cpc_CC_Actvn_Stat_PT : Outport  Description=|  Port=2
      | CC_Actvn_Stat (Chassis) and
      | CC_Actvn_Stat_PT (Powertrain)
      | have the same source in CPC,
      | but driver model expects ..._PT signal name
      settings: AttributesFormatString=%<Description>
  cpc_PT_Rdy_Stat : Outport  Description=needed for lvs model  Port=3
      settings: AttributesFormatString=%<Description>
  ch_CC_HystSpd_Rq_ICUC : Outport  Port=4
  ch_CC_LowHystSpd_Rq_ICUC : Outport  Port=5
  ch_CstValIPPC_Rq : Outport  Description=needed for PPC  Port=6
      settings: AttributesFormatString=%<Description>
  ch_CurvSpd_Rq : Outport  Description=needed for PPC  Port=7
      settings: AttributesFormatString=%<Description>
  ch_DipHystSpd_Rq : Outport  Port=8
  ch_SelSpdUnit_Stat : Outport  Port=9
  ch_AirTempOutsd_Cval_SCA : Outport  Port=10
  wires:
  convert10/1 -> cpc_ActOffCond_Stat/1  "cpc_ActOffCond_Stat"
  ActOffCond_Stat/1 -> convert10/1
  convert9/1 -> ch_CurvSpd_Rq/1  "ch_CurvSpd_Rq"
  drv_CurvSpd_Rq/1 -> convert9/1
  convert8/1 -> ch_CstValIPPC_Rq/1  "ch_CstValIPPC_Rq"
  drv_CstValIPPC_Rq/1 -> convert8/1
  convert7/1 -> cpc_PT_Rdy_Stat/1  "cpc_PT_Rdy_Stat"
  ch_PT_Rdy_Stat/1 -> convert7/1
  ch_CC_Actvn_Stat/1 -> convert5/1
  convert5/1 -> cpc_CC_Actvn_Stat_PT/1  "cpc_CC_Actvn_Stat_PT"
  drv_CC_LowHystSpd_Rq_ICUC/1 -> convert2/1
  drv_CC_HystSpd_Rq_ICUC/1 -> convert1/1
  convert1/1 -> ch_CC_HystSpd_Rq_ICUC/1  "ch_CC_HystSpd_Rq_ICUC"
  convert2/1 -> ch_CC_LowHystSpd_Rq_ICUC/1  "ch_CC_LowHystSpd_Rq_ICUC"
  convert3/1 -> ch_AirTempOutsd_Cval_SCA/1  "ch_AirTempOutsd_Cval_SCA"
  drv_DipHystSpd_Rq/1 -> convert6/1
  convert6/1 -> ch_DipHystSpd_Rq/1  "ch_DipHystSpd_Rq"
  convert4/1 -> ch_SelSpdUnit_Stat/1  "ch_SelSpdUnit_Stat"
  drv_SelSpdUnit_Stat/1 -> convert4/1
  env_Temperature/1 -> convert3/1

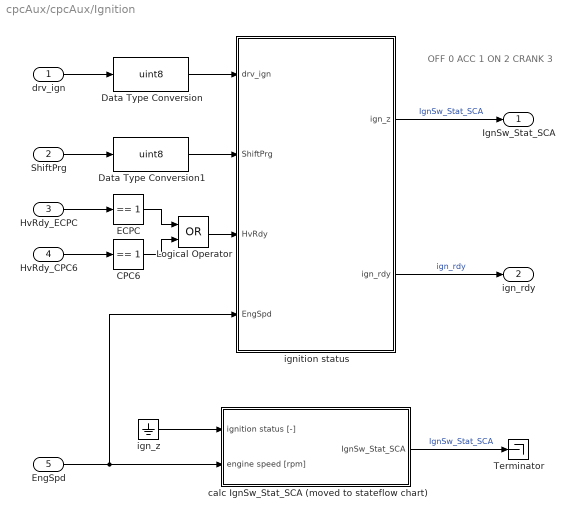
== system cpcAux/cpcAux/Ignition ==
  note: OFF	0
      | ACC 	1
      | ON   	2
      | CRANK	3
  drv_ign : Inport
  ShiftPrg : Inport  Port=2
  HvRdy_ECPC : Inport  Port=3
  HvRdy_CPC6 : Inport  Port=4
  EngSpd : Inport  Port=5
  CPC6 : simulink/Logic and Bit Operations/Compare To Constant  relop===  const=1  OutDataTypeStr=boolean
  Data Type Conversion : DataTypeConversion  OutDataTypeStr=uint8
  Data Type Conversion1 : DataTypeConversion  OutDataTypeStr=uint8
  ECPC : simulink/Logic and Bit Operations/Compare To Constant  relop===  const=1  OutDataTypeStr=boolean
  Logical Operator : Logic  Operator=OR  AllPortsSameDT=off  OutDataTypeStr=boolean
  Terminator : Terminator
  calc IgnSw_Stat_SCA (moved to stateflow chart) : Subsystem  mask{mdl_e_n_idle=500}
      mask prompts: mdl_e_n_idle "combustionEngine_idleSpeed_rpm"
  ign_z : Ground
  "ignition status " : Stateflow chart  TreatAsAtomicUnit=on
  IgnSw_Stat_SCA : Outport
  ign_rdy : Outport  Port=2
  wires:
  Data Type Conversion1/1 -> "ignition status "/2(ShiftPrg)
  CPC6/1 -> Logical Operator/2
  ECPC/1 -> Logical Operator/1
  ShiftPrg/1 -> Data Type Conversion1/1
  Logical Operator/1 -> "ignition status "/3(HvRdy)
  HvRdy_CPC6/1 -> CPC6/1
  HvRdy_ECPC/1 -> ECPC/1
  Data Type Conversion/1 -> "ignition status "/1(drv_ign)
  drv_ign/1 -> Data Type Conversion/1
  "ignition status "/2(ign_rdy) -> ign_rdy/1  "ign_rdy"
  calc IgnSw_Stat_SCA (moved to stateflow chart)/1(IgnSw_Stat_SCA) -> Terminator/1  "IgnSw_Stat_SCA"
  ign_z/1 -> calc IgnSw_Stat_SCA (moved to stateflow chart)/1(ignition status [-])
  "ignition status "/1(ign_z) -> IgnSw_Stat_SCA/1  "IgnSw_Stat_SCA"
  EngSpd/1 -> calc IgnSw_Stat_SCA (moved to stateflow chart)/2(engine speed [rpm]), "ignition status "/4(EngSpd)

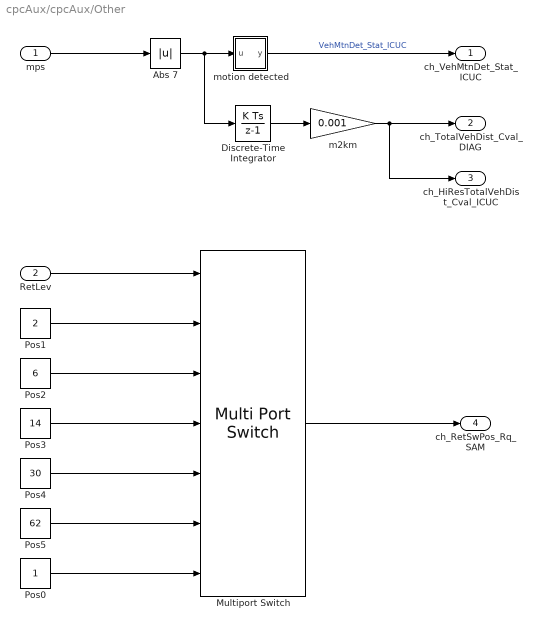
== system cpcAux/cpcAux/Other ==
  mps : Inport
  RetLev : Inport  Port=2
  Abs 7 : Abs
  Discrete-Time Integrator : DiscreteIntegrator  gainval=1  InitialConditionSetting=State (most efficient)  SampleTime=-1  ICPrevOutput=DiscIntNeverNeededParam  ICPrevScaledInput=DiscIntNeverNeededParam
  Multiport Switch : MultiPortSwitch  Inputs=5  DataPortForDefault=Additional data port  DiagnosticForDefault=None  OutDataTypeStr=double
      settings: AttributesFormatString=%<OutDataTypeStr>
  Pos0 : Constant
  Pos1 : Constant  Value=2
  Pos2 : Constant  Value=6
  Pos3 : Constant  Value=14
  Pos4 : Constant  Value=30
  Pos5 : Constant  Value=62
  m2km : Gain  Gain=0.001
  motion detected : Subsystem  mask(Compare To Constant){relop=>, const=0.5, OutDataTypeStr=uint8, ZeroCross=off}
      mask prompts: relop "Simulink:masks:Operator_MP"; const "Simulink:masks:ConstantValue_MP"; OutDataTypeStr "Simulink:masks:OutputDataType_MP"; ZeroCross "Simulink:masks:EnableZerocrossingDetection_MP"
      mask help: Simulink:masks:CompareToConstant_MD
      mask init:
      | blkName = gcb;
      | 
      | if strcmp(get_param(gcbh,'OutDataTypeStr'),'boolean')
      | 	setValue = 'boolean';
      | else
      | 	setValue = 'fixdt(0, 8)';
      | end
      | 
      | set_param([blkName,'/Compare'],'relop',relop, ...
      | 	'OutDataTypeStr', setValue, 'ZeroCross', ZeroCross);
      | 
      | str = [relop,' C']; %default
      | 
      | const_str = get_param(blkName, 'const');
      | 
      | if isempty(strfind(const_str, ' ')) && isempty(strfind(const_str, ','))
      |     % scalar or single expression
      |     if isempty(str2num(const_str))
      |         %expression
      |         str = [relop, ' ', const_str];
      |     elseif length(const) == 1
      |         str = [relop,' ',num2str(double(const))];
      |     end
      | end
      mask TypeOptions relop: == | ~= | < | <= | >= | >
      mask TypeOptions OutDataTypeStr: Simulink:masks:uint8 | Simulink:masks:boolean
      mask Callback ZeroCross: sl('zeroCrossEnable', gcbh);
      mask Display: disp(str)
  ch_VehMtnDet_Stat_ICUC : Outport
  ch_TotalVehDist_Cval_DIAG : Outport  Port=2
  ch_HiResTotalVehDist_Cval_ICUC : Outport  Port=3
  ch_RetSwPos_Rq_SAM : Outport  Port=4
  wires:
  Multiport Switch/1 -> ch_RetSwPos_Rq_SAM/1
  Pos0/1 -> Multiport Switch/7
  Pos5/1 -> Multiport Switch/6
  Pos4/1 -> Multiport Switch/5
  Pos3/1 -> Multiport Switch/4
  Pos2/1 -> Multiport Switch/3
  Pos1/1 -> Multiport Switch/2
  RetLev/1 -> Multiport Switch/1
  Discrete-Time Integrator/1 -> m2km/1
  m2km/1 -> ch_TotalVehDist_Cval_DIAG/1, ch_HiResTotalVehDist_Cval_ICUC/1
  motion detected/1(y) -> ch_VehMtnDet_Stat_ICUC/1  "VehMtnDet_Stat_ICUC"
  Abs 7/1 -> motion detected/1(u), Discrete-Time Integrator/1
  mps/1 -> Abs 7/1

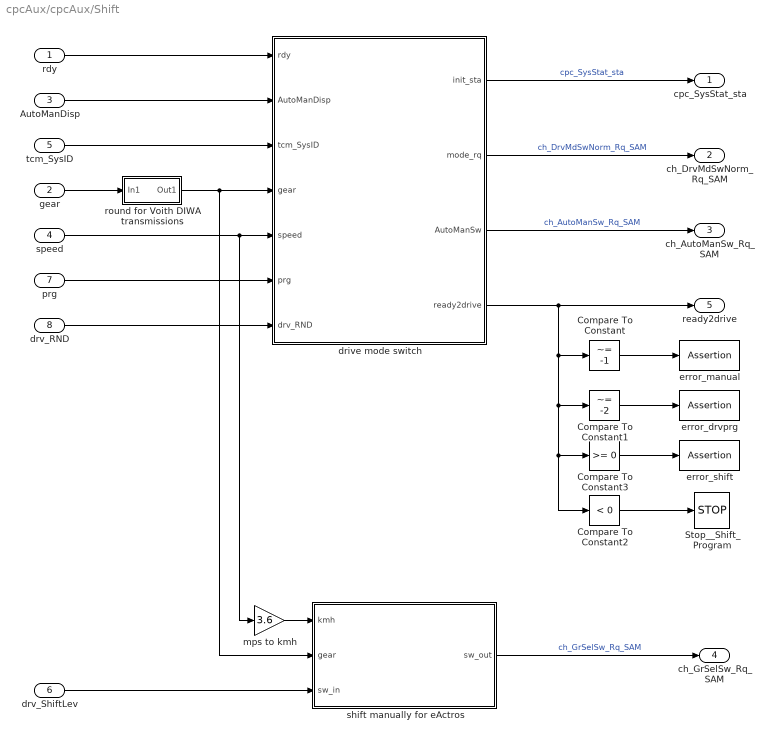
== system cpcAux/cpcAux/Shift ==
  rdy : Inport
  gear : Inport  Port=2
  AutoManDisp : Inport  Port=3
  speed : Inport  Port=4
  tcm_SysID : Inport  Port=5
  drv_ShiftLev : Inport  Port=6
  prg : Inport  Port=7
  drv_RND : Inport  Port=8
  Compare To Constant : simulink/Logic and Bit Operations/Compare To Constant  relop=~=  const=-1  OutDataTypeStr=boolean
  Compare To Constant1 : simulink/Logic and Bit Operations/Compare To Constant  relop=~=  const=-2  OutDataTypeStr=boolean
  Compare To Constant2 : simulink/Logic and Bit Operations/Compare To Constant  relop=<  const=0  OutDataTypeStr=boolean
  Compare To Constant3 : simulink/Logic and Bit Operations/Compare To Constant  relop=>=  const=0  OutDataTypeStr=boolean
  Stop__Shift_Program : Stop  Description=The simulation completes the current time step before terminating
      settings: AttributesFormatString=%<Description>
  drive mode switch : Stateflow chart  TreatAsAtomicUnit=on
  error_drvprg : Assertion  AssertionFailFcn=fprintf(2,'cpcAux: Drive Program is not accepted by CPC\n')  StopWhenAssertionFail=off
  error_manual : Assertion  AssertionFailFcn=fprintf(2,'cpcAux: vehicle stays in automatic\n')  StopWhenAssertionFail=off
  error_shift : Assertion  AssertionFailFcn=fprintf(2,'cpcAux: Error in Shift, abort simulation\n')  StopWhenAssertionFail=off
  mps to kmh : Gain  Gain=3.6
  round for Voith DIWA transmissions : Subsystem  Description=|  mask(Round){resolution=1e-6}
      | gear values are not exactly integer values all the time,
      | probably due to some numerical calculation reasons
      mask help: Round values to defined resolution
      mask Display: disp(resolution)
  shift manually for eActros : Subsystem
  cpc_SysStat_sta : Outport
  ch_DrvMdSwNorm_Rq_SAM : Outport  Port=2
  ch_AutoManSw_Rq_SAM : Outport  Port=3
  ch_GrSelSw_Rq_SAM : Outport  Port=4
  ready2drive : Outport  Port=5
  wires:
  rdy/1 -> drive mode switch/1(rdy)
  drv_RND/1 -> drive mode switch/7(drv_RND)
  round for Voith DIWA transmissions/1(Out1) -> drive mode switch/4(gear), shift manually for eActros/2(gear)
  Compare To Constant1/1 -> error_drvprg/1
  prg/1 -> drive mode switch/6(prg)
  Compare To Constant/1 -> error_manual/1
  AutoManDisp/1 -> drive mode switch/2(AutoManDisp)
  drive mode switch/3(AutoManSw) -> ch_AutoManSw_Rq_SAM/1  "ch_AutoManSw_Rq_SAM"
  mps to kmh/1 -> shift manually for eActros/1(kmh)
  shift manually for eActros/1(sw_out) -> ch_GrSelSw_Rq_SAM/1  "ch_GrSelSw_Rq_SAM"
  drv_ShiftLev/1 -> shift manually for eActros/3(sw_in)
  tcm_SysID/1 -> drive mode switch/3(tcm_SysID)
  drive mode switch/1(init_sta) -> cpc_SysStat_sta/1  "cpc_SysStat_sta"
  drive mode switch/2(mode_rq) -> ch_DrvMdSwNorm_Rq_SAM/1  "ch_DrvMdSwNorm_Rq_SAM"
  gear/1 -> round for Voith DIWA transmissions/1(In1)
  speed/1 -> drive mode switch/5(speed), mps to kmh/1
  Compare To Constant2/1 -> Stop__Shift_Program/1
  drive mode switch/4(ready2drive) -> ready2drive/1, Compare To Constant/1, Compare To Constant2/1, Compare To Constant3/1, Compare To Constant1/1
  Compare To Constant3/1 -> error_shift/1

== system cpcAux/cpcAux/Transfer Gear Box ==
  transfer case state : Stateflow chart  TreatAsAtomicUnit=on
  DiffLkIAC_Stat : Outport
  SFA_Ind_Stat : Outport  Port=2
  TrfGrBoxRng_Stat : Outport  Port=3
  wires:
  transfer case state/1(InterAxleDrfLock) -> DiffLkIAC_Stat/1  "CGW.EAC1_SCH.DiffLkIAC_Stat"
  transfer case state/2(FrontAxleEng) -> SFA_Ind_Stat/1  "CGW.SCH_E1.SFA_Ind_Stat"
  transfer case state/3(TrfGboxGear) -> TrfGrBoxRng_Stat/1  "CGW.SCH_E1.TrfGrBoxRng_Stat"

== system cpcAux/cpcAux/eActros Drivertrain ready ==
  rdy : Inport
  ch_PT_Rdy_Stat : Inport  Port=2
  Active : simulink/Logic and Bit Operations/Compare To Constant  relop===  const=1  OutDataTypeStr=boolean
  Constant : Constant  OutDataTypeStr=boolean
  Manual Switch : ManualSwitch
  PT Ready Check : Subsystem  TreatAsAtomicUnit=on
  SNA : simulink/Logic and Bit Operations/Compare To Constant  relop===  const=3  OutDataTypeStr=boolean
  and : Logic  AllPortsSameDT=off  OutDataTypeStr=boolean
  or : Logic  Operator=OR  AllPortsSameDT=off  OutDataTypeStr=boolean
  drivetrain_rdy : Outport
  wires:
  Manual Switch/1 -> drivetrain_rdy/1, PT Ready Check/1(PT_ready)
  Constant/1 -> Manual Switch/2
  and/1 -> Manual Switch/1
  rdy/1 -> and/1, PT Ready Check/Enable
  ch_PT_Rdy_Stat/1 -> Active/1, SNA/1
  or/1 -> and/2
  Active/1 -> or/1
  SNA/1 -> or/2

== system cpcAux/cpcAux/Blinds/Referenzierung scharf schalten ==
  Constant : Constant  Value=3
  Constant1 : Constant  Value=0
  Digital Clock : DigitalClock  SampleTime=-1
  Switch : Switch  Criteria=u2 ~= 0
  Wrap To Zero after 3 s : simulink/Discontinuities/Wrap To Zero  Threshold=3
  ActMovStat : Outport
  wires:
  Switch/1 -> ActMovStat/1
  Wrap To Zero after 3 s/1 -> Switch/2
  Constant/1 -> Switch/1
  Constant1/1 -> Switch/3
  Digital Clock/1 -> Wrap To Zero after 3 s/1

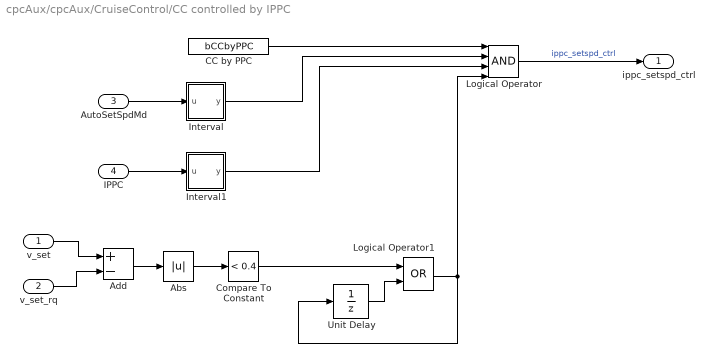
== system cpcAux/cpcAux/CruiseControl/CC controlled by IPPC ==
  v_set : Inport
  v_set_rq : Inport  Port=2
  AutoSetSpdMd : Inport  Port=3
  IPPC : Inport  Port=4
  Abs : Abs
  Add : Sum  Inputs=+-
  CC by PPC : Constant  Value=bCCbyPPC
  Compare To Constant : simulink/Logic and Bit Operations/Compare To Constant  relop=<  const=0.4  OutDataTypeStr=boolean
  Interval : Subsystem  mask(Interval Test){IntervalClosedRight=on, uplimit=2, IntervalClosedLeft=on, lowlimit=1, OutDataTypeStr=boolean}
      mask prompts: IntervalClosedRight "Simulink:masks:IntervalClosedOnRight_MP"; uplimit "Simulink:masks:UpperLimit_MP"; IntervalClosedLeft "Simulink:masks:IntervalClosedOnLeft_MP"; lowlimit "Simulink:masks:LowerLimit_MP"; OutDataTypeStr "Simulink:masks:OutputDataType_MP"
      mask help: Simulink:masks:IntervalTest_MD
      mask init:
      | if IntervalClosedLeft
      |   lOff = 0;
      |   lRelop = '<=';
      | else
      |   lOff = 0.1;
      |   lRelop = '<';
      | end
      | if IntervalClosedRight
      |   rOff = 0;
      |   uRelop = '<=';
      | else
      |   rOff = 0.1;
      |   uRelop = '<';
      | end
      | 
      | blkH = gcbh;
      | blkName = getfullname(blkH);
      | 
      | set_param([blkName,'/Upper Test'],'relop',uRelop);
      | set_param([blkName,'/Lower Test'],'relop',lRelop);
      | if strcmp(get_param(blkH,'OutDataTypeStr'),'boolean')
      | set_param([blkName,'/AND'],'OutDataTypeStr','boolean');
      | else
      | set_param([blkName,'/AND'],'OutDataTypeStr','fixdt(0, 8)');
      | end
      settings: AttributesFormatString=%<lowlimit> ... %<uplimit>
      mask TypeOptions OutDataTypeStr: Simulink:masks:uint8 | Simulink:masks:boolean
      mask Display: plot([0 1],[0.3 0.3],[0.3 0.3],[0 1],[0 0.2 0.2],[0.35 0.35 0.55-lOff],[0.2 0.2 0.55 0.55],[0.55+lOff 0.75 0.75 0.55+rOff],[0.55 0.55 1],[0.55-rOff 0.35 0.35]);
  Interval1 : Subsystem  mask(Interval Test){IntervalClosedRight=on, uplimit=3, IntervalClosedLeft=on, lowlimit=1, OutDataTypeStr=boolean}
      mask prompts: IntervalClosedRight "Simulink:masks:IntervalClosedOnRight_MP"; uplimit "Simulink:masks:UpperLimit_MP"; IntervalClosedLeft "Simulink:masks:IntervalClosedOnLeft_MP"; lowlimit "Simulink:masks:LowerLimit_MP"; OutDataTypeStr "Simulink:masks:OutputDataType_MP"
      mask help: Simulink:masks:IntervalTest_MD
      mask init: same as cpcAux/cpcAux/CruiseControl/CC controlled by IPPC/Interval
      settings: AttributesFormatString=%<lowlimit> ... %<uplimit>
      mask TypeOptions OutDataTypeStr: Simulink:masks:uint8 | Simulink:masks:boolean
      mask Display: plot([0 1],[0.3 0.3],[0.3 0.3],[0 1],[0 0.2 0.2],[0.35 0.35 0.55-lOff],[0.2 0.2 0.55 0.55],[0.55+lOff 0.75 0.75 0.55+rOff],[0.55 0.55 1],[0.55-rOff 0.35 0.35]);
  Logical Operator : Logic  Inputs=4  AllPortsSameDT=off  OutDataTypeStr=boolean
  Logical Operator1 : Logic  Operator=OR  AllPortsSameDT=off  OutDataTypeStr=boolean
  Unit Delay : UnitDelay  SampleTime=-1
  ippc_setspd_ctrl : Outport
  wires:
  Abs/1 -> Compare To Constant/1
  Add/1 -> Abs/1
  v_set_rq/1 -> Add/2
  Logical Operator1/1 -> Logical Operator/4, Unit Delay/1
  Unit Delay/1 -> Logical Operator1/2
  Compare To Constant/1 -> Logical Operator1/1
  v_set/1 -> Add/1
  Interval1/1(y) -> Logical Operator/3
  Interval/1(y) -> Logical Operator/2
  AutoSetSpdMd/1 -> Interval/1(u)
  IPPC/1 -> Interval1/1(u)
  CC by PPC/1 -> Logical Operator/1
  Logical Operator/1 -> ippc_setspd_ctrl/1  "ippc_setspd_ctrl"

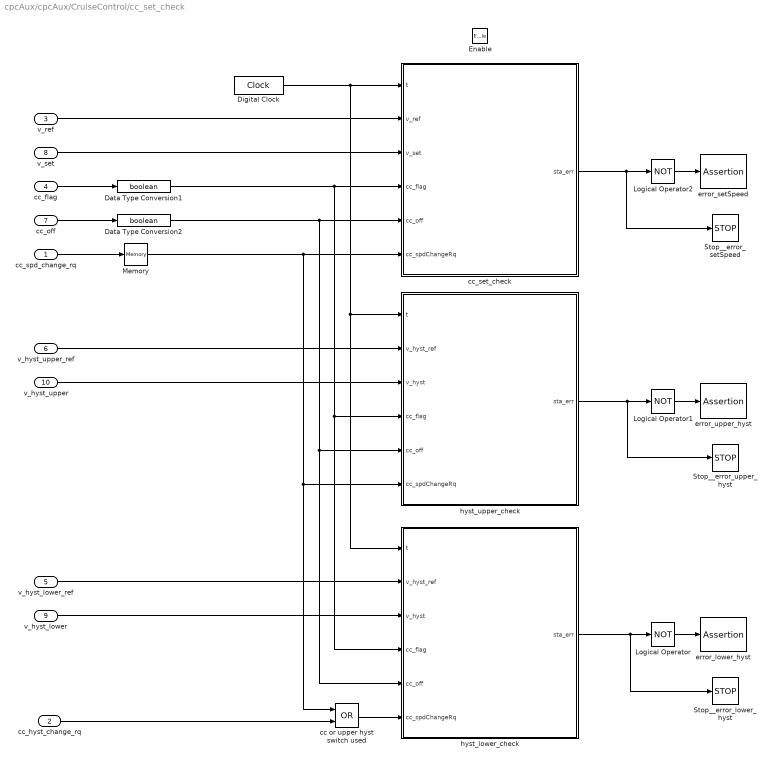
== system cpcAux/cpcAux/CruiseControl/cc_set_check ==
  cc_spd_change_rq : Inport
  cc_hyst_change_rq : Inport  Port=2
  v_ref : Inport  Port=3
  cc_flag : Inport  Port=4
  v_hyst_lower_ref : Inport  Port=5
  v_hyst_upper_ref : Inport  Port=6
  cc_off : Inport  Port=7
  v_set : Inport  Port=8
  v_hyst_lower : Inport  Port=9
  v_hyst_upper : Inport  Port=10
  Enable : EnablePort
  Data Type Conversion1 : DataTypeConversion  OutDataTypeStr=boolean
  Data Type Conversion2 : DataTypeConversion  OutDataTypeStr=boolean
  Digital Clock : DigitalClock  SampleTime=-1
  Logical Operator : Logic  Operator=NOT  AllPortsSameDT=off  OutDataTypeStr=boolean
  Logical Operator1 : Logic  Operator=NOT  AllPortsSameDT=off  OutDataTypeStr=boolean
  Logical Operator2 : Logic  Operator=NOT  AllPortsSameDT=off  OutDataTypeStr=boolean
  Memory : Memory  InheritSampleTime=on
  Stop__error_lower_hyst : Stop  Description=The simulation completes the current time step before terminating
      settings: AttributesFormatString=%<Description>
  Stop__error_setSpeed : Stop  Description=The simulation completes the current time step before terminating
      settings: AttributesFormatString=%<Description>
  Stop__error_upper_hyst : Stop  Description=The simulation completes the current time step before terminating
      settings: AttributesFormatString=%<Description>
  cc or upper hyst switch used : Logic  Operator=OR  AllPortsSameDT=off  OutDataTypeStr=boolean
  cc_set_check : Stateflow chart  TreatAsAtomicUnit=on
  error_lower_hyst : Assertion  AssertionFailFcn=fprintf(2,'cpcAux: DRV request of lower CC hysteresis is not accepted by CPC \n')  StopWhenAssertionFail=off
  error_setSpeed : Assertion  AssertionFailFcn=fprintf(2,'cpcAux: DRV request of set speed is not accepted by CPC \n')  StopWhenAssertionFail=off
  error_upper_hyst : Assertion  AssertionFailFcn=fprintf(2,'cpcAux: DRV request of upper CC hysteresis is not accepted by CPC \n')  StopWhenAssertionFail=off
  hyst_lower_check : Stateflow chart  TreatAsAtomicUnit=on
  hyst_upper_check : Stateflow chart  TreatAsAtomicUnit=on
  wires:
  cc or upper hyst switch used/1 -> hyst_lower_check/6(cc_spdChangeRq)
  cc_hyst_change_rq/1 -> cc or upper hyst switch used/2
  Memory/1 -> cc or upper hyst switch used/1, hyst_upper_check/6(cc_spdChangeRq), cc_set_check/6(cc_spdChangeRq)
  Data Type Conversion1/1 -> hyst_lower_check/4(cc_flag), hyst_upper_check/4(cc_flag), cc_set_check/4(cc_flag)
  cc_off/1 -> Data Type Conversion2/1
  cc_set_check/1(sta_err) -> Logical Operator2/1, Stop__error_setSpeed/1
  Logical Operator2/1 -> error_setSpeed/1
  v_ref/1 -> cc_set_check/2(v_ref)
  cc_spd_change_rq/1 -> Memory/1
  v_set/1 -> cc_set_check/3(v_set)
  Data Type Conversion2/1 -> hyst_lower_check/5(cc_off), hyst_upper_check/5(cc_off), cc_set_check/5(cc_off)
  v_hyst_upper/1 -> hyst_upper_check/3(v_hyst)
  v_hyst_upper_ref/1 -> hyst_upper_check/2(v_hyst_ref)
  hyst_upper_check/1(sta_err) -> Logical Operator1/1, Stop__error_upper_hyst/1
  Logical Operator1/1 -> error_upper_hyst/1
  hyst_lower_check/1(sta_err) -> Logical Operator/1, Stop__error_lower_hyst/1
  Logical Operator/1 -> error_lower_hyst/1
  Digital Clock/1 -> hyst_lower_check/1(t), hyst_upper_check/1(t), cc_set_check/1(t)
  v_hyst_lower_ref/1 -> hyst_lower_check/2(v_hyst_ref)
  v_hyst_lower/1 -> hyst_lower_check/3(v_hyst)
  cc_flag/1 -> Data Type Conversion1/1

== system cpcAux/cpcAux/CruiseControl/cc_spd_change_req ==
  cc_spd_inc : Inport
  cc_spc_dec : Inport  Port=2
  cc_hyst_inc : Inport  Port=3
  cc_hyst_dec : Inport  Port=4
  Logical Operator : Logic  Operator=OR  AllPortsSameDT=off  OutDataTypeStr=boolean
  Logical Operator1 : Logic  Operator=OR  AllPortsSameDT=off  OutDataTypeStr=boolean
  cc_spd_change : Outport
  cc_hyst_change : Outport  Port=2
  wires:
  Logical Operator1/1 -> cc_hyst_change/1
  cc_hyst_dec/1 -> Logical Operator1/2
  cc_hyst_inc/1 -> Logical Operator1/1
  cc_spc_dec/1 -> Logical Operator/2
  cc_spd_inc/1 -> Logical Operator/1
  Logical Operator/1 -> cc_spd_change/1

== system cpcAux/cpcAux/CruiseControl/kmh_round ==
  note: round to defined resolution
  In1 : Inport
  Constant : Constant  Value=1/resolution
      settings: AttributesFormatString=%<Value>
  Divide : Product  Inputs=*/
  Gain : Gain  Gain=3.6
      settings: AttributesFormatString=%<Gain>
  Product : Product
  Rounding Function : Rounding  Operator=round
  Out1 : Outport
  wires:
  In1/1 -> Gain/1
  Gain/1 -> Product/1
  Divide/1 -> Out1/1
  Rounding Function/1 -> Divide/1
  Product/1 -> Rounding Function/1
  Constant/1 -> Product/2, Divide/2

== system cpcAux/cpcAux/DateTime/SNA1 ==
  In : Inport
  Constant : Constant  Value=sna_eq
  Switch : Switch  Criteria=u2 > Threshold  Threshold=sna_max
  Out : Outport
  wires:
  In/1 -> Switch/3, Switch/2
  Switch/1 -> Out/1
  Constant/1 -> Switch/1

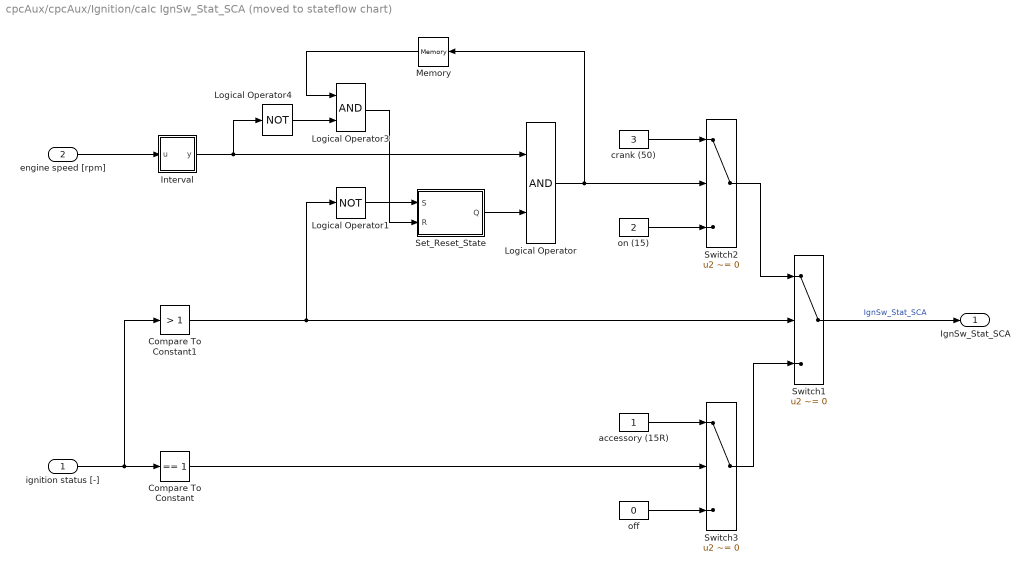
== system cpcAux/cpcAux/Ignition/calc IgnSw_Stat_SCA (moved to stateflow chart) ==
  ignition status [-] : Inport
  engine speed [rpm] : Inport  Port=2
  Compare To Constant : simulink/Logic and Bit Operations/Compare To Constant  relop===  const=1  OutDataTypeStr=boolean
  Compare To Constant1 : simulink/Logic and Bit Operations/Compare To Constant  relop=>  const=1  OutDataTypeStr=boolean
  Interval : Subsystem  mask(Interval Test){IntervalClosedRight=on, uplimit=mdl_e_n_idle - 200, IntervalClosedLeft=on, lowlimit=20, OutDataTypeStr=boolean}
      mask prompts: IntervalClosedRight "Simulink:masks:IntervalClosedOnRight_MP"; uplimit "Simulink:masks:UpperLimit_MP"; IntervalClosedLeft "Simulink:masks:IntervalClosedOnLeft_MP"; lowlimit "Simulink:masks:LowerLimit_MP"; OutDataTypeStr "Simulink:masks:OutputDataType_MP"
      mask help: Simulink:masks:IntervalTest_MD
      mask init: same as cpcAux/cpcAux/CruiseControl/CC controlled by IPPC/Interval
      settings: AttributesFormatString=[%<lowlimit> rpm - (%<uplimit>) rpm]
      mask TypeOptions OutDataTypeStr: Simulink:masks:uint8 | Simulink:masks:boolean
      mask Display: plot([0 1],[0.3 0.3],[0.3 0.3],[0 1],[0 0.2 0.2],[0.35 0.35 0.55-lOff],[0.2 0.2 0.55 0.55],[0.55+lOff 0.75 0.75 0.55+rOff],[0.55 0.55 1],[0.55-rOff 0.35 0.35]);
  Logical Operator : Logic  OutDataTypeStr=boolean
  Logical Operator1 : Logic  Operator=NOT  OutDataTypeStr=boolean
  Logical Operator3 : Logic  OutDataTypeStr=boolean
  Logical Operator4 : Logic  Operator=NOT  OutDataTypeStr=boolean
  Memory : Memory  InheritSampleTime=on
  Set_Reset_State : Subsystem  mask(SRFlipFlop){initial_condition=0, t=-1}
      mask prompts: initial_condition "Initial condition (state of Q):"; t "Sampletime (-1 for inherited)"
      mask help: S-R Flip-Flop Block
      mask Help:
      | The S-R flip-flop also known as a set-reset flip-flop. This implementation
      | is modeled after an S-R flip-flop constructed using NOR gates. The
      | truth table for this block is:
      | <pre>
      |  S  R   Q  !Q
      |  ----------------
      |  1  0   1  0
      |  0  0   1  0  (after S == 1, R == 0)
      |  0  1   0  1
      |  0  0   0  1  (after S == 0, R == 1)
      |  1  1   0  0
      | </pre>
      | 
      | In an S-R flip-flop that is implemented with NOR gates, when a 1 is
      | applied to both the set and reset inputs, both outputs go to 0. Technically,
      | this state is undefined and is usually avoided. Note, if the flip-flop is
      | implemented with NAND gates, when a 0 is applied to both inputs, both outputs
      | go to 0 and when a 1 is applied to both inputs, the output depends on
      | the previous state of the flip-flop (previous value of Q).
  Switch1 : Switch  Criteria=u2 ~= 0  Threshold=0.5  InputSameDT=on
      settings: AttributesFormatString=%<Criteria>
  Switch2 : Switch  Criteria=u2 ~= 0  Threshold=0.5  InputSameDT=on
      settings: AttributesFormatString=%<Criteria>
  Switch3 : Switch  Criteria=u2 ~= 0  Threshold=0.5  InputSameDT=on
      settings: AttributesFormatString=%<Criteria>
  accessory (15R) : Constant  OutDataTypeStr=uint8
  crank (50) : Constant  Value=3  OutDataTypeStr=uint8
  off : Constant  Value=0  OutDataTypeStr=uint8
  on (15) : Constant  Value=2  OutDataTypeStr=uint8
  IgnSw_Stat_SCA : Outport
  wires:
  accessory (15R)/1 -> Switch3/1
  Switch3/1 -> Switch1/3
  off/1 -> Switch3/3
  Compare To Constant/1 -> Switch3/2
  Logical Operator1/1 -> Set_Reset_State/1(S)
  Logical Operator4/1 -> Logical Operator3/2
  Logical Operator3/1 -> Set_Reset_State/2(R)
  Logical Operator/1 -> Switch2/2, Memory/1
  Set_Reset_State/1(Q) -> Logical Operator/2
  Interval/1(y) -> Logical Operator4/1, Logical Operator/1
  crank (50)/1 -> Switch2/1
  on (15)/1 -> Switch2/3
  Switch2/1 -> Switch1/1
  Switch1/1 -> IgnSw_Stat_SCA/1  "IgnSw_Stat_SCA"
  Compare To Constant1/1 -> Logical Operator1/1, Switch1/2
  ignition status [-]/1 -> Compare To Constant/1, Compare To Constant1/1
  engine speed [rpm]/1 -> Interval/1(u)
  Memory/1 -> Logical Operator3/1
